simulink model "nmwtest"  (Simulink 9.1)
settings: Solver=VariableStepDiscrete  StartTime=0.0  StopTime=nmwtest_param.endTime  RelTol=1e-3  EnableMultiTasking=on
PreLoadFcn:
  | % Run the setup script when the model is opened
  | setup_nmwtest;
InitFcn:
  | % Run the setup script again just before the
  | % model is run, so that any updates made
  | % after opening are applied.
  | setup_nmwtest;
undefined symbols (not defined in the file or in its folder): nmwtest_param, value
libraries: DSPBABase x6, simulink x4, DSPBAFilters x1, DSPBAPrim x1
Description:
  | DSP Builder Advanced Template for Template Design implementing ModelIP designs
settings Model: Creator=mjervis  LastModifiedBy=klutc_000
settings DataIOCC: LimitDataPoints=on  SignalLoggingSaveFormat=ModelDataLogs
settings OptimizationCC: ExpressionDepthLimit=2147483647
settings DebuggingCC: SolverPrmCheckMsg=warning  InheritedTsInSrcMsg=none  IntegerOverflowMsg=none  FcnCallInpInsideContextMsg=warning  StateNameClashWarn=warning  IntegerSaturationMsg=none
settings GRTTargetCC: GeneratePreprocessorConditionals=Disable all

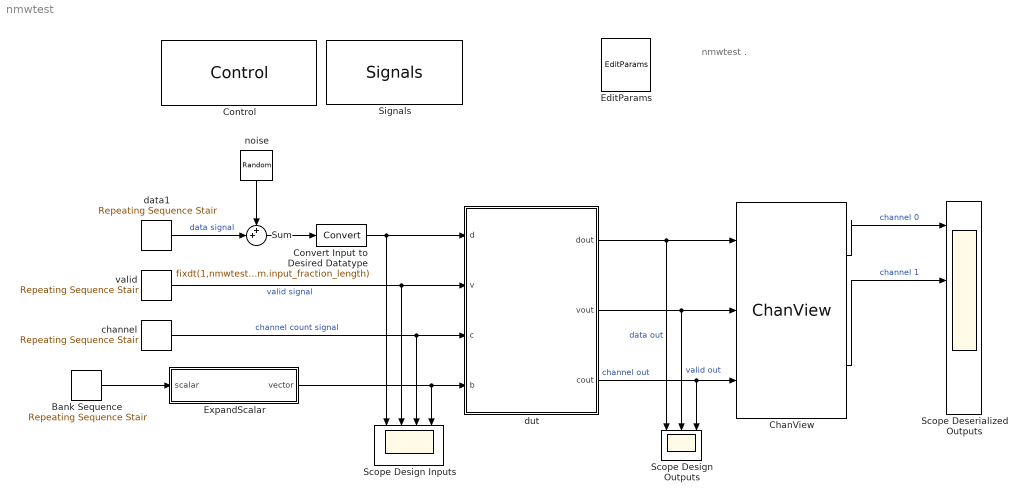
== system nmwtest ==
  note: nmwtest
      |                                          .
  Bank Sequence : simulink/Sources/Repeating Sequence Stair  OutValues=[ones(1,nmwtest_param.Period*100) zeros(1,nmwtest_param.Period*100)]  tsamp=nmwtest_param.SampleTime  OutMin=[]  OutMax=[]  OutDataTypeStr=Inherit: Inherit via back propagation  OutDataType=float('double')  ConRadixGroup=Best Precision: Vector-wise  OutScaling=2^-12
  ChanView : DSPBABase/ChanView  nchans=nmwtest_param.ChanCount  chan_vector=[0:nmwtest_param.ChanCount-1]  outsvalid=off  latency=1  version=20090407
  Control : DSPBABase/Control  generate=on  language=VHDL  destination=./rtl  destination_gui=./rtl  make_full_path=off  quartus_work=../rtl  quartus_work_gui=../rtl  path_is_relative=on  autotestbench=on  signaldepth=2  coveragetestbench=off  logs=off  spacewidth=2  spacenum=1  addrwidth=10  datawidth=16  dataendian=Big Endian  hierarchicalnames=off  ramThresholdBits=-1  distRamThresholdBits=-1  mlabThresholdBits=-1  hardMultiplierThresholdLuts=-1  version=20090407  errorOnChanMismatch=on  errorOnGPIOMismatch=off  importModelsimResults=0  floatMismatchTolerance=-1.0  floatMismatchZeroTolerance=-1.0  cycleAccurate=off  reinterpretCastMult=off  paramFile=nmwtest_params.xml
  Convert Input to Desired Datatype : DataTypeConversion  OutDataTypeStr=fixdt(1,nmwtest_param.input_word_length,nmwtest_param.input_fraction_length)  SaturateOnIntegerOverflow=on
  EditParams : DSPBABase/EditParams  version=20090407
  ExpandScalar : Subsystem  mask{vecWidth=nmwtest_param.ChanWireCount}
      mask prompts: vecWidth "Vector Width"
      mask help:
      | Take a single, scalar connection and replicate it to form a vector of duplicate signals.
      |
      | This is an auto-generating masked subsystem built from primitive (ModelPrim) blocks.
      |
      | Right click on the block and select 'Look Under Mask' to see the structure or View Mask, Initialization tab to see the generation commands.
      mask init:
      | set_param(gcb, 'MaskSelfModifiable', 'on');
      | delete_line(find_system(gcb, 'SearchDepth', 1,...
      |             'FollowLinks', 'on', 'LookUnderMasks', 'all',...
      |             'FindAll', 'on', 'Type', 'line'));
      | if ~isempty(find_system(gcb, 'SearchDepth', 1,...
      |             'FollowLinks', 'on', 'LookUnderMasks', 'all',...
      |             'Name', 'Mux'))
      |         delete_block([gcb '/Mux']);
      | end
      | 
      | add_block('built-in/Mux', [gcb '/Mux'], 'Inputs', int2str(vecWidth), 'DisplayOption', 'bar');
      | 
      | for n=1:vecWidth
      |     add_line(gcb, 'scalar/1', sprintf('Mux/%d', n));
      | end
      | add_line(gcb, 'Mux/1', 'vector/1');
      mask Display:
      | color('w');
      | image(imread('dspba_prim_masked.png'));
      | fprintf('expand\nscalar');
      | port_label('input',1,'scalar');
      | port_label('output',1,'vector');
  Scope Deserialized Outputs : Scope  NumInputPorts=4
  Scope Design Inputs : Scope  NumInputPorts=4
  Scope Design Outputs : Scope  NumInputPorts=3
  Signals : DSPBABase/Signals  clk=clk  freq=nmwtest_param.ClockRate  margin=nmwtest_param.ClockMargin  rst=areset  rstactive=High  bus=bus  enbusclock=off  busfreq=62.5  bussync=off  version=20090407
  Sum : Sum  Inputs=++|
  channel : simulink/Sources/Repeating Sequence Stair  OutValues=[0:nmwtest_param.ChanCycleCount-1 zeros(1,nmwtest_param.Period-nmwtest_param.ChanCycleCount)]  tsamp=nmwtest_param.SampleTime  OutMin=[]  OutMax=[]  OutDataTypeStr=uint8  OutputDataTypeScalingMode=uint8  OutDataType=uint8  ConRadixGroup=Best Precision: Vector-wise  OutScaling=2^-12
  data1 : simulink/Sources/Repeating Sequence Stair  OutValues=[0 0.5 1]  tsamp=nmwtest_param.SampleTime  OutMin=[]  OutMax=[]  OutDataTypeStr=Inherit: Inherit via back propagation  OutDataType=fixdt('sfix16_En15')  ConRadixGroup=Best Precision: Vector-wise  OutScaling=[]
  dut : Subsystem
  noise : UniformRandomNumber  Minimum=-0.125  Maximum=0.125  Seed=0:nmwtest_param.ChanWireCount-1  SampleTime=nmwtest_param.SampleTime
  valid : simulink/Sources/Repeating Sequence Stair  OutValues=[ones(1,nmwtest_param.ChanCycleCount) zeros(1,nmwtest_param.Period-nmwtest_param.ChanCycleCount)]  tsamp=nmwtest_param.SampleTime  OutMin=[]  OutMax=[]  OutDataTypeStr=Inherit: Inherit via back propagation  OutDataType=fixdt(0,1,0)  ConRadixGroup=Best Precision: Vector-wise  OutScaling=[]
  wires:
  dut/2(vout) -> ChanView/2, Scope Design Outputs/2  "valid out"
  dut/3(cout) -> ChanView/3, Scope Design Outputs/3  "channel out"
  dut/1(dout) -> ChanView/1, Scope Design Outputs/1  "data out"
  valid/1 -> dut/2(v), Scope Design Inputs/2  "valid signal"
  channel/1 -> dut/3(c), Scope Design Inputs/3  "channel count signal"
  Convert Input to Desired Datatype/1 -> dut/1(d), Scope Design Inputs/1
  ChanView/1 -> Scope Deserialized Outputs/1  "channel 0"
  ChanView/2 -> Scope Deserialized Outputs/2  "channel 1"
  ? -> Scope Deserialized Outputs/3  "channel 2"
  ? -> Scope Deserialized Outputs/4  "channel 3"
  data1/1 -> Sum/2  "data signal"
  noise/1 -> Sum/1
  Sum/1 -> Convert Input to Desired Datatype/1
  Bank Sequence/1 -> ExpandScalar/1(scalar)
  ExpandScalar/1(vector) -> dut/4(b), Scope Design Inputs/4

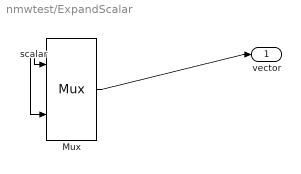
== system nmwtest/ExpandScalar ==
  scalar : Inport
  Mux : Mux  Inputs=2
  vector : Outport
  wires:
  scalar/1 -> Mux/1, Mux/2
  Mux/1 -> vector/1

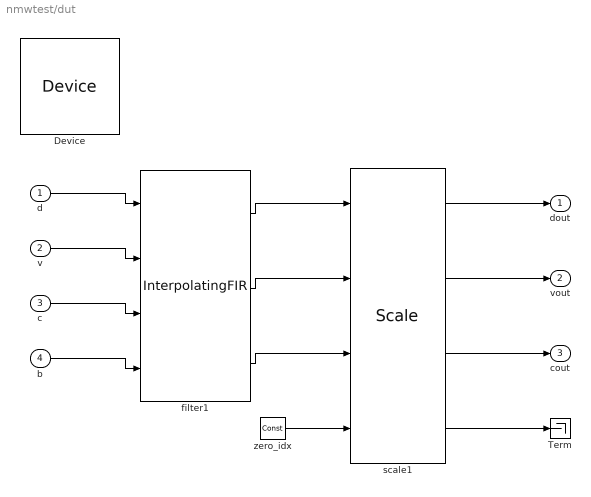
== system nmwtest/dut ==
  d : Inport
  v : Inport  Port=2
  c : Inport  Port=3
  b : Inport  Port=4
  Device : DSPBABase/Device  family=Stratix IV  deviceMember=Stratix IV GX  stratix4device=Stratix IV GX  hardcopy4device=HardCopy IV E  stratix5device=Stratix V GX  device=AUTO  speed=-2  stratixSpeed=-5  stratix2Speed=-3  stratix3Speed=-3  stratix4gxSpeed=-2  stratix4gtSpeed=-1  cyclone2Speed=-6  cyclone3Speed=-7  arria2Speed=-4  cyclone4eSpeed=-8  stratix5Speed=-3  arria5Speed=-4  arriaSpeed=-6  cyclone3lsSpeed=-7  cyclone5Speed=-6  arria2gzSpeed=-3  nightFurySpeed=-2  ecp2Speed=-7  hardcopycompat=off  version=20140217  max10flashmode=off  max10nomeminit=off
  Term : Terminator
  filter1 : DSPBAFilters/InterpolatingFIR  nInputRate=nmwtest_param.filter1.SampleRate  interp=nmwtest_param.filter1.Interpolation  nchan=nmwtest_param.ChanCount  symmetry=Symmetrical  coef=nmwtest_param.filter1.coeffs  addr=nmwtest_param.filter1.base_addr  rwmode=Write  nband=Use All Taps  exposebus=off  latency=6  version=20090407  recon=off  MM=[0,1,2,3,4,5,6,7,8,9,10,11,12,13,14,15]
  scale1 : DSPBABase/Scale  otype=sfix(nmwtest_param.output_word_length)  scale=2^-nmwtest_param.output_fraction_length  rndmethod=Truncate  factor=1  satmethod=None  shift_vec=0  latency=0  wideSimulation=off  version=20090407
  zero_idx : DSPBAPrim/Const  primtype=const  nInputs=0  nOutputs=1  omode=Inherit via internal rule  otype=sfix(16)  scale=2^-15  rndmethod=Unbiased  factor=1  satmethod=Symmetric  shift_vec=[0 1 2 -1]  value=0  inPortNames=['+'; '+';]  outPortNames=[' ']  dspbaimage=dspba_prim.jpg  text=fprintf('%s', num2str(value));  style=Optimised  visibilities=8 + 1024  floatPrecision=float32_m23  version=20120820
  dout : Outport
  vout : Outport  Port=2
  cout : Outport  Port=3
  wires:
  d/1 -> filter1/1
  v/1 -> filter1/2
  filter1/2 -> scale1/2
  c/1 -> filter1/3
  filter1/3 -> scale1/3
  filter1/1 -> scale1/1
  b/1 -> filter1/4
  scale1/1 -> dout/1
  scale1/2 -> vout/1
  scale1/3 -> cout/1
  zero_idx/1 -> scale1/4
  scale1/4 -> Term/1
